simulink model "Comp_Output_Wrapper"  (R2020b)
settings: configuration reference "VLS_Standard_RH850" (kept outside this file)
undefined symbols (not defined in the file): C_EndIndexOfEachLightingModule, C_IsDrlPlOnTps, C_IsTiOnTps, C_StartIndexOfEachLightingModule, N_CONST_100, N_CONST_NULL, N_PowerSupply2
libraries: simulink x6
settings Model: DataDictionary=New_SLDD.sldd  Creator=ahashem  LastModifiedBy=ahashem
settings ConfigSetRef: SourceName=VLS_Standard_RH850

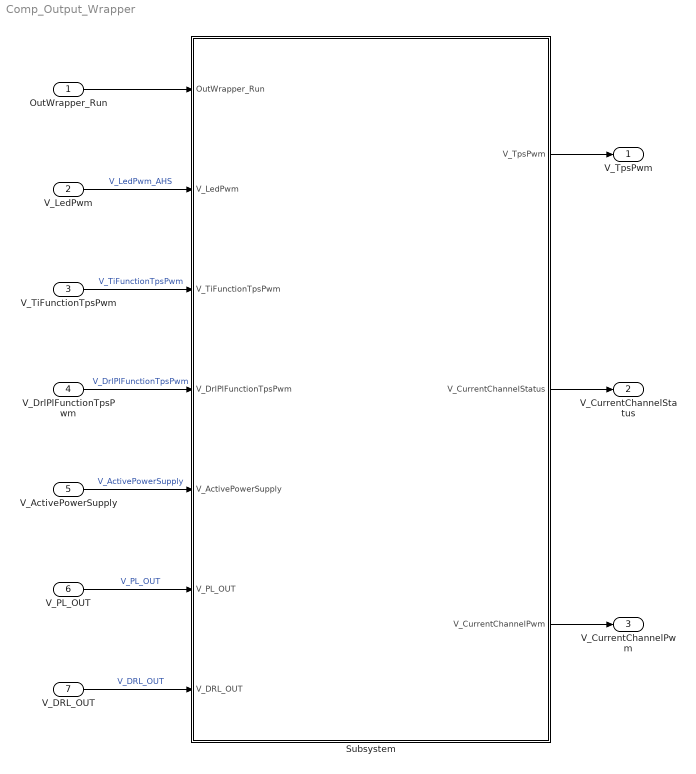
== system Comp_Output_Wrapper ==
  OutWrapper_Run : Inport  OutputFunctionCall=on
  V_LedPwm : Inport  Port=2
  V_TiFunctionTpsPwm : Inport  Port=3
  V_DrlPlFunctionTpsPwm : Inport  Port=4
  V_ActivePowerSupply : Inport  Port=5
  V_PL_OUT : Inport  Port=6
  V_DRL_OUT : Inport  Port=7
  Subsystem : Subsystem
  V_TpsPwm : Outport
  V_CurrentChannelStatus : Outport  Port=2
  V_CurrentChannelPwm : Outport  Port=3
  wires:
  OutWrapper_Run/1 -> Subsystem/1(OutWrapper_Run)
  V_TiFunctionTpsPwm/1 -> Subsystem/3(V_TiFunctionTpsPwm)  "V_TiFunctionTpsPwm"
  V_DrlPlFunctionTpsPwm/1 -> Subsystem/4(V_DrlPlFunctionTpsPwm)  "V_DrlPlFunctionTpsPwm"
  V_ActivePowerSupply/1 -> Subsystem/5(V_ActivePowerSupply)  "V_ActivePowerSupply"
  V_LedPwm/1 -> Subsystem/2(V_LedPwm)  "V_LedPwm_AHS"
  V_PL_OUT/1 -> Subsystem/6(V_PL_OUT)  "V_PL_OUT"
  V_DRL_OUT/1 -> Subsystem/7(V_DRL_OUT)  "V_DRL_OUT"
  Subsystem/1(V_TpsPwm) -> V_TpsPwm/1
  Subsystem/2(V_CurrentChannelStatus) -> V_CurrentChannelStatus/1
  Subsystem/3(V_CurrentChannelPwm) -> V_CurrentChannelPwm/1

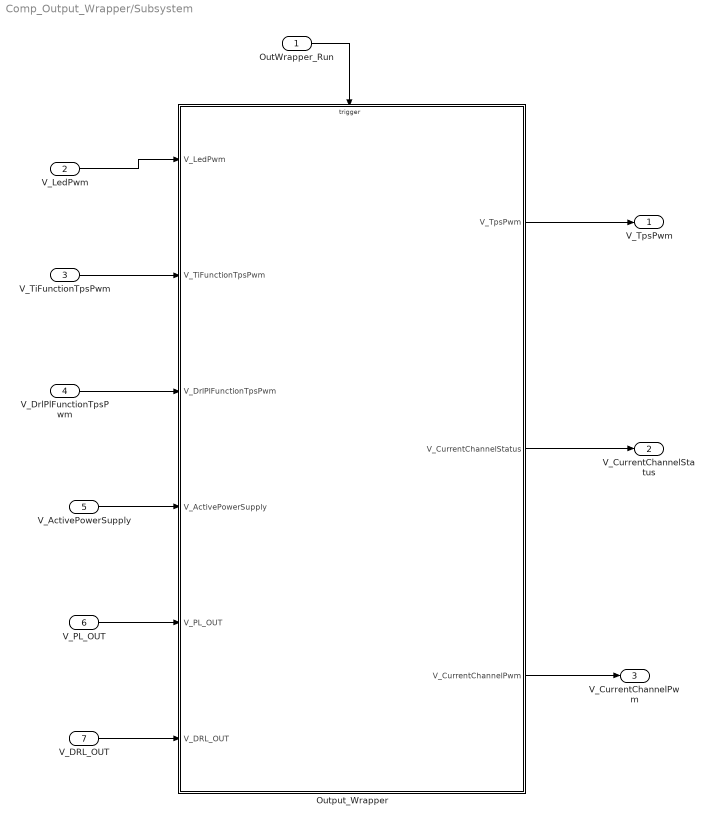
== system Comp_Output_Wrapper/Subsystem ==
  OutWrapper_Run : Inport
  V_LedPwm : Inport  Port=2
  V_TiFunctionTpsPwm : Inport  Port=3
  V_DrlPlFunctionTpsPwm : Inport  Port=4
  V_ActivePowerSupply : Inport  Port=5
  V_PL_OUT : Inport  Port=6
  V_DRL_OUT : Inport  Port=7
  Output_Wrapper : Subsystem
  V_TpsPwm : Outport
  V_CurrentChannelStatus : Outport  Port=2
  V_CurrentChannelPwm : Outport  Port=3
  wires:
  V_TiFunctionTpsPwm/1 -> Output_Wrapper/2(V_TiFunctionTpsPwm)
  V_DrlPlFunctionTpsPwm/1 -> Output_Wrapper/3(V_DrlPlFunctionTpsPwm)
  V_PL_OUT/1 -> Output_Wrapper/5(V_PL_OUT)
  V_LedPwm/1 -> Output_Wrapper/1(V_LedPwm)
  V_ActivePowerSupply/1 -> Output_Wrapper/4(V_ActivePowerSupply)
  V_DRL_OUT/1 -> Output_Wrapper/6(V_DRL_OUT)
  OutWrapper_Run/1 -> Output_Wrapper/Trigger
  Output_Wrapper/1(V_TpsPwm) -> V_TpsPwm/1
  Output_Wrapper/2(V_CurrentChannelStatus) -> V_CurrentChannelStatus/1
  Output_Wrapper/3(V_CurrentChannelPwm) -> V_CurrentChannelPwm/1

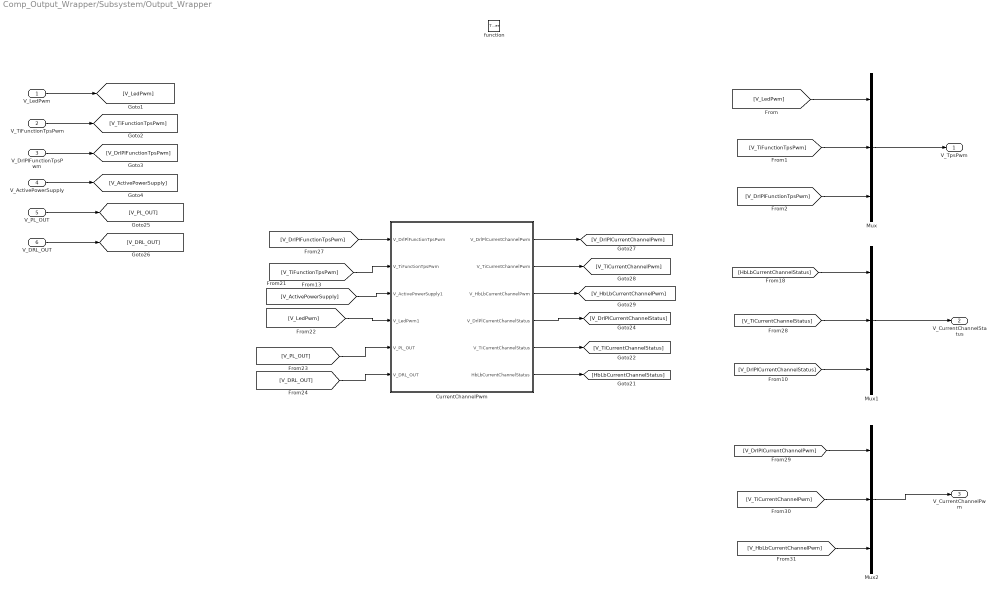
== system Comp_Output_Wrapper/Subsystem/Output_Wrapper ==
  V_LedPwm : Inport
  V_TiFunctionTpsPwm : Inport  Port=2
  V_DrlPlFunctionTpsPwm : Inport  Port=3
  V_ActivePowerSupply : Inport  Port=4
  V_PL_OUT : Inport  Port=5
  V_DRL_OUT : Inport  Port=6
  function : TriggerPort  TriggerType=function-call  VariantControl=Variant
  CurrentChannelPwm : Subsystem
  Mux : Mux  Inputs=3
  Mux1 : Mux  Inputs=3
  Mux2 : Mux  Inputs=3
  V_TpsPwm : Outport
  V_CurrentChannelStatus : Outport  Port=2
  V_CurrentChannelPwm : Outport  Port=3
  wires:
  [V_DRL_OUT] -> CurrentChannelPwm/6(V_DRL_OUT)
  [HbLbCurrentChannelStatus] -> Mux1/1
  CurrentChannelPwm/4(V_DrlPlCurrentChannelStatus) -> [V_DrlPlCurrentChannelStatus]
  V_LedPwm/1 -> [V_LedPwm]
  [V_LedPwm] -> CurrentChannelPwm/4(V_LedPwm1)
  Mux/1 -> V_TpsPwm/1
  [V_DrlPlFunctionTpsPwm] -> CurrentChannelPwm/1(V_DrlPlFunctionTpsPwm)
  V_DRL_OUT/1 -> [V_DRL_OUT]
  CurrentChannelPwm/2(V_TiCurrentChannelPwm) -> [V_TiCurrentChannelPwm]
  Mux2/1 -> V_CurrentChannelPwm/1
  [V_ActivePowerSupply] -> CurrentChannelPwm/3(V_ActivePowerSupply1)
  CurrentChannelPwm/3(V_HbLbCurrentChannelPwm) -> [V_HbLbCurrentChannelPwm]
  [V_DrlPlCurrentChannelStatus] -> Mux1/3
  [V_HbLbCurrentChannelPwm] -> Mux2/3
  Mux1/1 -> V_CurrentChannelStatus/1
  [V_PL_OUT] -> CurrentChannelPwm/5(V_PL_OUT)
  [V_DrlPlCurrentChannelPwm] -> Mux2/1
  [V_TiCurrentChannelStatus] -> Mux1/2
  V_TiFunctionTpsPwm/1 -> [V_TiFunctionTpsPwm]
  CurrentChannelPwm/6(HbLbCurrentChannelStatus) -> [HbLbCurrentChannelStatus]
  V_DrlPlFunctionTpsPwm/1 -> [V_DrlPlFunctionTpsPwm]
  V_ActivePowerSupply/1 -> [V_ActivePowerSupply]
  CurrentChannelPwm/5(V_TiCurrentChannelStatus) -> [V_TiCurrentChannelStatus]
  V_PL_OUT/1 -> [V_PL_OUT]
  [V_TiFunctionTpsPwm] -> CurrentChannelPwm/2(V_TiFunctionTpsPwm)
  CurrentChannelPwm/1(V_DrlPlCurrentChannelPwm) -> [V_DrlPlCurrentChannelPwm]
  [V_DrlPlFunctionTpsPwm] -> Mux/3
  [V_TiCurrentChannelPwm] -> Mux2/2
  [V_LedPwm] -> Mux/1
  [V_TiFunctionTpsPwm] -> Mux/2

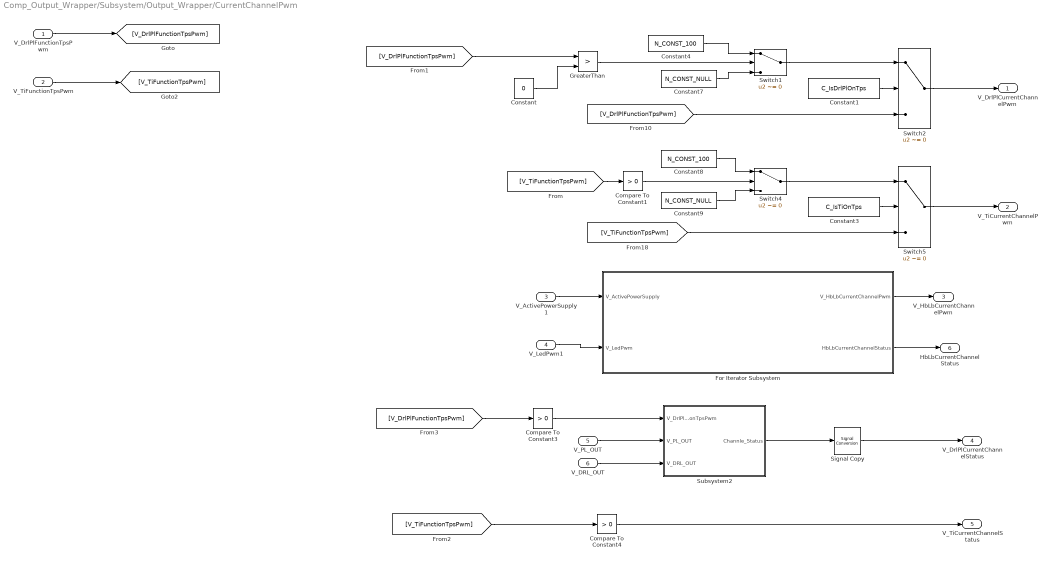
== system Comp_Output_Wrapper/Subsystem/Output_Wrapper/CurrentChannelPwm ==
  V_DrlPlFunctionTpsPwm : Inport
  V_TiFunctionTpsPwm : Inport  Port=2
  V_ActivePowerSupply1 : Inport  Port=3
  V_LedPwm1 : Inport  Port=4
  V_PL_OUT : Inport  Port=5
  V_DRL_OUT : Inport  Port=6
  Compare To Constant1 : simulink/Logic and Bit Operations/Compare To Constant  relop=>  const=0  OutDataTypeStr=boolean
  Compare To Constant3 : simulink/Logic and Bit Operations/Compare To Constant  relop=>  const=0  OutDataTypeStr=boolean
  Compare To Constant4 : simulink/Logic and Bit Operations/Compare To Constant  relop=>  const=0  OutDataTypeStr=boolean
  Constant : Constant  Value=0  OutDataTypeStr=Inherit: Inherit via back propagation
  Constant1 : Constant  Value=C_IsDrlPlOnTps
  Constant3 : Constant  Value=C_IsTiOnTps
  Constant4 : Constant  Value=N_CONST_100  OutDataTypeStr=Inherit: Inherit via back propagation
  Constant7 : Constant  Value=N_CONST_NULL  OutDataTypeStr=Inherit: Inherit via back propagation
  Constant8 : Constant  Value=N_CONST_100  OutDataTypeStr=Inherit: Inherit via back propagation
  Constant9 : Constant  Value=N_CONST_NULL  OutDataTypeStr=Inherit: Inherit via back propagation
  For Iterator Subsystem : Subsystem  TreatAsAtomicUnit=on
  GreaterThan : RelationalOperator  Operator=>  OutDataTypeStr=boolean  RndMeth=Simplest
  Signal Copy : SignalConversion  OverrideOpt=off
  Subsystem2 : Subsystem
  Switch1 : Switch  Criteria=u2 ~= 0  OutDataTypeStr=Inherit: Inherit via back propagation
  Switch2 : Switch  Criteria=u2 ~= 0
  Switch4 : Switch  Criteria=u2 ~= 0  OutDataTypeStr=Inherit: Inherit via back propagation
  Switch5 : Switch  Criteria=u2 ~= 0
  V_DrlPlCurrentChannelPwm : Outport
  V_TiCurrentChannelPwm : Outport  Port=2
  V_HbLbCurrentChannelPwm : Outport  Port=3
  V_DrlPlCurrentChannelStatus : Outport  Port=4
  V_TiCurrentChannelStatus : Outport  Port=5
  HbLbCurrentChannelStatus : Outport  Port=6
  wires:
  [V_DrlPlFunctionTpsPwm] -> GreaterThan/1
  Constant/1 -> GreaterThan/2
  Constant1/1 -> Switch2/2
  [V_DrlPlFunctionTpsPwm] -> Switch2/3
  Constant4/1 -> Switch1/1
  Switch1/1 -> Switch2/1
  Switch2/1 -> V_DrlPlCurrentChannelPwm/1
  GreaterThan/1 -> Switch1/2
  Constant3/1 -> Switch5/2
  Compare To Constant1/1 -> Switch4/2
  [V_TiFunctionTpsPwm] -> Switch5/3
  Switch4/1 -> Switch5/1
  Constant8/1 -> Switch4/1
  Constant9/1 -> Switch4/3
  Constant7/1 -> Switch1/3
  Switch5/1 -> V_TiCurrentChannelPwm/1
  V_DrlPlFunctionTpsPwm/1 -> [V_DrlPlFunctionTpsPwm]
  V_LedPwm1/1 -> For Iterator Subsystem/2(V_LedPwm)
  V_ActivePowerSupply1/1 -> For Iterator Subsystem/1(V_ActivePowerSupply)
  For Iterator Subsystem/1(V_HbLbCurrentChannelPwm) -> V_HbLbCurrentChannelPwm/1
  Compare To Constant4/1 -> V_TiCurrentChannelStatus/1
  Signal Copy/1 -> V_DrlPlCurrentChannelStatus/1
  [V_TiFunctionTpsPwm] -> Compare To Constant4/1
  Compare To Constant3/1 -> Subsystem2/1(V_DrlPlFunctionTpsPwm)
  V_PL_OUT/1 -> Subsystem2/2(V_PL_OUT)
  Subsystem2/1(Channle_Status) -> Signal Copy/1
  [V_DrlPlFunctionTpsPwm] -> Compare To Constant3/1
  V_DRL_OUT/1 -> Subsystem2/3(V_DRL_OUT)
  For Iterator Subsystem/2(HbLbCurrentChannelStatus) -> HbLbCurrentChannelStatus/1
  V_TiFunctionTpsPwm/1 -> [V_TiFunctionTpsPwm]
  [V_TiFunctionTpsPwm] -> Compare To Constant1/1

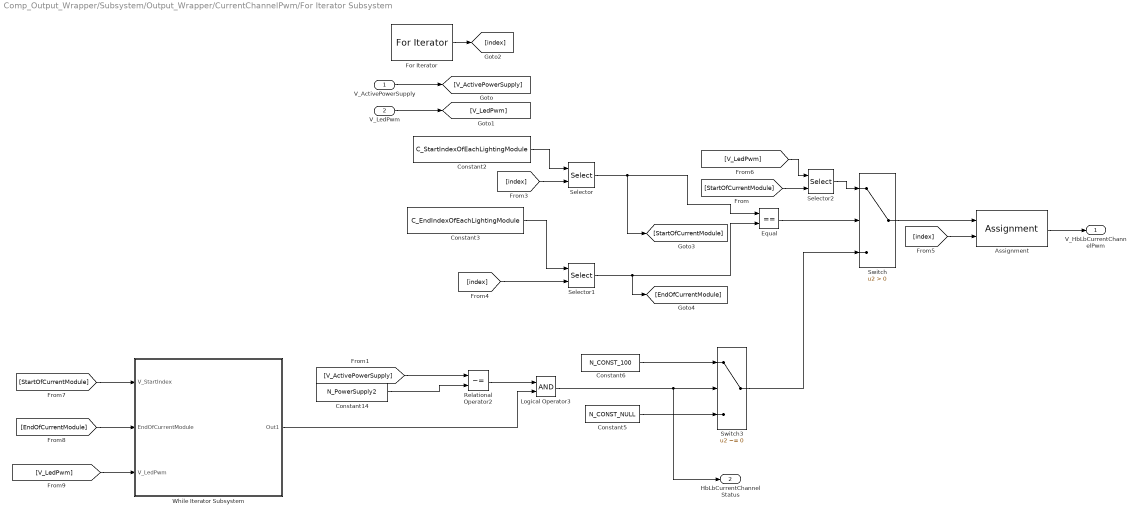
== system Comp_Output_Wrapper/Subsystem/Output_Wrapper/CurrentChannelPwm/For Iterator Subsystem ==
  V_ActivePowerSupply : Inport
  V_LedPwm : Inport  Port=2
  Assignment : Assignment  IndexMode=Zero-based  OutputInitialize=Specify size for each dimension in table  DiagnosticForDimensions=Error  IndexOptions=Starting index (port)  Indices=1  OutputSizes=1
  Constant14 : Constant  Value=N_PowerSupply2  OutDataTypeStr=Inherit: Inherit via back propagation
  Constant2 : Constant  Value=C_StartIndexOfEachLightingModule
  Constant3 : Constant  Value=C_EndIndexOfEachLightingModule
  Constant5 : Constant  Value=N_CONST_NULL
  Constant6 : Constant  Value=N_CONST_100  OutDataTypeStr=Inherit: Inherit via back propagation
  Equal : RelationalOperator  Operator===  OutDataTypeStr=boolean  RndMeth=Simplest
  For Iterator : ForIterator  IterationLimit=C_NumOfLightingModules  IndexMode=Zero-based
  Logical Operator3 : Logic  AllPortsSameDT=off  OutDataTypeStr=boolean
  Relational Operator2 : RelationalOperator  Operator=~=  OutDataTypeStr=boolean  RndMeth=Simplest
  Selector : Selector  IndexMode=Zero-based  InputPortWidth=3  IndexOptions=Index vector (port)  Indices=[1 3]  OutputSizes=1
  Selector1 : Selector  IndexMode=Zero-based  IndexOptions=Index vector (port)  Indices=[1 3]  OutputSizes=1
  Selector2 : Selector  IndexMode=Zero-based  IndexOptions=Index vector (port)  Indices=[1 3]  OutputSizes=1
  Switch : Switch  Criteria=u2 > Threshold
  Switch3 : Switch  Criteria=u2 ~= 0
  While Iterator Subsystem : Subsystem  TreatAsAtomicUnit=on
  V_HbLbCurrentChannelPwm : Outport
  HbLbCurrentChannelStatus : Outport  Port=2
  wires:
  Selector/1 -> [StartOfCurrentModule], Equal/1
  Selector1/1 -> [EndOfCurrentModule], Equal/2
  Equal/1 -> Switch/2
  V_ActivePowerSupply/1 -> [V_ActivePowerSupply]
  V_LedPwm/1 -> [V_LedPwm]
  Selector2/1 -> Switch/1
  Constant14/1 -> Relational Operator2/2
  Constant6/1 -> Switch3/1
  Switch3/1 -> Switch/3
  Relational Operator2/1 -> Logical Operator3/1
  Constant5/1 -> Switch3/3
  Logical Operator3/1 -> HbLbCurrentChannelStatus/1, Switch3/2
  While Iterator Subsystem/1(Out1) -> Logical Operator3/2
  [V_ActivePowerSupply] -> Relational Operator2/1
  Switch/1 -> Assignment/1
  For Iterator/1 -> [index]
  [index] -> Selector/2
  [index] -> Selector1/2
  Constant2/1 -> Selector/1
  Constant3/1 -> Selector1/1
  Assignment/1 -> V_HbLbCurrentChannelPwm/1
  [index] -> Assignment/2
  [V_LedPwm] -> Selector2/1
  [StartOfCurrentModule] -> Selector2/2
  [StartOfCurrentModule] -> While Iterator Subsystem/1(V_StartIndex)
  [EndOfCurrentModule] -> While Iterator Subsystem/2(EndOfCurrentModule)
  [V_LedPwm] -> While Iterator Subsystem/3(V_LedPwm)

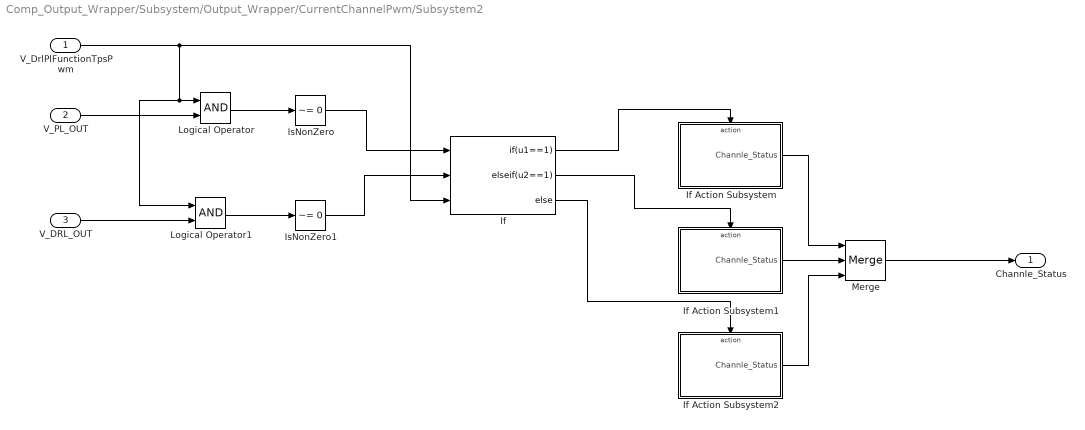
== system Comp_Output_Wrapper/Subsystem/Output_Wrapper/CurrentChannelPwm/Subsystem2 ==
  V_DrlPlFunctionTpsPwm : Inport
  V_PL_OUT : Inport  Port=2
  V_DRL_OUT : Inport  Port=3
  If : If  NumInputs=3  IfExpression=u1==1  ElseIfExpressions=u2==1
  If Action Subsystem : Subsystem  TreatAsAtomicUnit=on
  If Action Subsystem1 : Subsystem  TreatAsAtomicUnit=on
  If Action Subsystem2 : Subsystem  TreatAsAtomicUnit=on
  IsNonZero : simulink/Logic and Bit Operations/Compare To Zero  relop=~=  OutDataTypeStr=boolean
  IsNonZero1 : simulink/Logic and Bit Operations/Compare To Zero  relop=~=  OutDataTypeStr=boolean
  Logical Operator : Logic  AllPortsSameDT=off  OutDataTypeStr=boolean
  Logical Operator1 : Logic  AllPortsSameDT=off  OutDataTypeStr=boolean
  Merge : Merge  Inputs=3
  Channle_Status : Outport
  wires:
  V_PL_OUT/1 -> Logical Operator/2
  If/1 -> If Action Subsystem/Action
  Merge/1 -> Channle_Status/1
  V_DrlPlFunctionTpsPwm/1 -> If/3, Logical Operator1/1, Logical Operator/1
  If/2 -> If Action Subsystem1/Action
  Logical Operator1/1 -> IsNonZero1/1
  IsNonZero/1 -> If/1
  If/3 -> If Action Subsystem2/Action
  V_DRL_OUT/1 -> Logical Operator1/2
  If Action Subsystem2/1(Channle_Status) -> Merge/3
  Logical Operator/1 -> IsNonZero/1
  If Action Subsystem/1(Channle_Status) -> Merge/1
  IsNonZero1/1 -> If/2
  If Action Subsystem1/1(Channle_Status) -> Merge/2

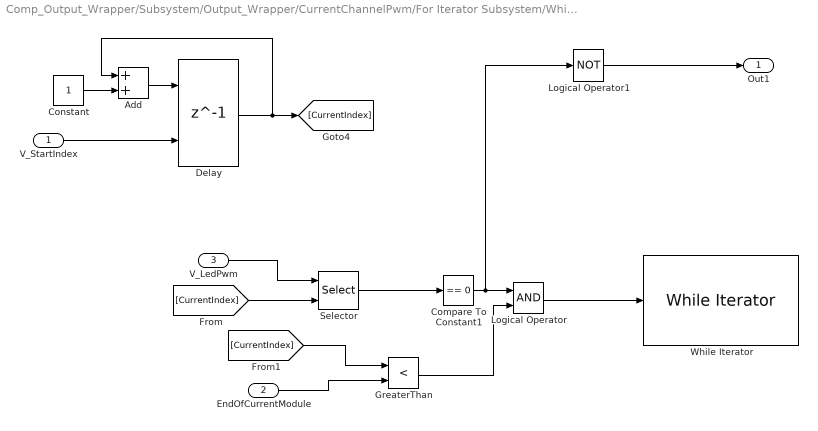
== system Comp_Output_Wrapper/Subsystem/Output_Wrapper/CurrentChannelPwm/For Iterator Subsystem/While Iterator Subsystem ==
  V_StartIndex : Inport
  EndOfCurrentModule : Inport  Port=2
  V_LedPwm : Inport  Port=3
  Add : Sum  AccumDataTypeStr=uint32  OutDataTypeStr=uint32
  Compare To Constant1 : simulink/Logic and Bit Operations/Compare To Constant  relop===  const=0  OutDataTypeStr=boolean
  Constant : Constant  OutDataTypeStr=uint8
  Delay : Delay  DelayLength=1  InitialConditionSource=Input port
      settings: InputPortMap=u0,p4
  GreaterThan : RelationalOperator  Operator=<  OutDataTypeStr=boolean  RndMeth=Simplest
  Logical Operator : Logic  AllPortsSameDT=off  OutDataTypeStr=boolean
  Logical Operator1 : Logic  Operator=NOT  AllPortsSameDT=off  OutDataTypeStr=boolean
  Selector : Selector  IndexMode=Zero-based  IndexOptions=Index vector (port)  Indices=[1 3]  OutputSizes=1
  While Iterator : WhileIterator  MaxIters=-1  WhileBlockType=do-while
  Out1 : Outport
  wires:
  Compare To Constant1/1 -> Logical Operator1/1, Logical Operator/1
  V_StartIndex/1 -> Delay/2
  Add/1 -> Delay/1
  Delay/1 -> Add/1, [CurrentIndex]
  Constant/1 -> Add/2
  [CurrentIndex] -> Selector/2
  V_LedPwm/1 -> Selector/1
  Selector/1 -> Compare To Constant1/1
  [CurrentIndex] -> GreaterThan/1
  EndOfCurrentModule/1 -> GreaterThan/2
  GreaterThan/1 -> Logical Operator/2
  Logical Operator/1 -> While Iterator/1
  Logical Operator1/1 -> Out1/1

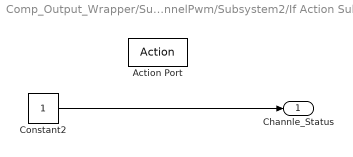
== system Comp_Output_Wrapper/Subsystem/Output_Wrapper/CurrentChannelPwm/Subsystem2/If Action Subsystem ==
  Action Port : ActionPort  ActionPortLabel=if(u1==1)
  Constant2 : Constant  OutDataTypeStr=Inherit: Inherit via back propagation
  Channle_Status : Outport
  wires:
  Constant2/1 -> Channle_Status/1

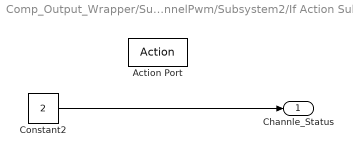
== system Comp_Output_Wrapper/Subsystem/Output_Wrapper/CurrentChannelPwm/Subsystem2/If Action Subsystem1 ==
  Action Port : ActionPort  ActionPortLabel=elseif(u2==1)
  Constant2 : Constant  Value=2  OutDataTypeStr=Inherit: Inherit via back propagation
  Channle_Status : Outport
  wires:
  Constant2/1 -> Channle_Status/1

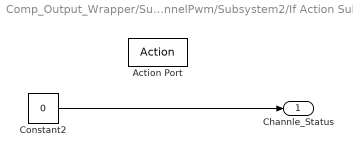
== system Comp_Output_Wrapper/Subsystem/Output_Wrapper/CurrentChannelPwm/Subsystem2/If Action Subsystem2 ==
  Action Port : ActionPort  ActionPortLabel=else
  Constant2 : Constant  Value=0  OutDataTypeStr=Inherit: Inherit via back propagation
  Channle_Status : Outport
  wires:
  Constant2/1 -> Channle_Status/1
